simulink model "simulering_ROV_DP_model2"  (R2020a)
settings: Solver=VariableStepAuto  StartTime=0.0  StopTime=t_sim  RelTol=1e-3
values from neighbouring files (symbols this model uses):
  B_aug = [b11 b12 b13 b14 b15 b16 ... (first row only)    [constants.m]
  B_psinv_aug = B_aug'/(B_aug*B_aug')    [constants.m]
  coriolis_effect = 1    [run_simulation.m]    (also in run_simulation_STA_controller.m; run_simulation_dp_model.m)
  d_11 = 250    [constants.m]    (also in constants_dp_model.m; constants_model_coriolis.m; constants_process_model.m)
  d_22 = 200    [constants.m]    (also in constants_dp_model.m; constants_model_coriolis.m; constants_process_model.m)
  d_33 = 175    [constants.m]    (also in constants_dp_model.m; constants_model_coriolis.m; constants_process_model.m)
  d_66 = 15    [constants.m]    (also in constants_process_model.m)
  d_n11 = 350    [constants.m]
  d_n22 = 350    [constants.m]
  d_n33 = 400    [constants.m]
  d_n66 = 75    [constants.m]
  Delta = 25    [plot_simulation_feedback.m]    (also in run_simulation.m; run_simulation_SM_controller.m; run_simulation_STA_controller.m; run_simulation_dp_model.m)
  g_z = 9.81    [run_simulation_FL_controller.m]    (also in run_simulation_PID_controller.m = 0.91; run_simulation_SM_controller.m = 0.91; run_simulation_STA_controller.m = 0.91; run_simulation_dp_model.m = 0.91)
  gamma1 = 50    [run_simulation_dp_model.m]    (also in tuning_dp_model.m = 5)
  gamma2 = 35    [run_simulation_dp_model.m]    (also in tuning_dp_model.m = 3.5)
  gamma_e1 = 0.05    [tuning_dp_model.m]
  gamma_e2 = 0.05    [tuning_dp_model.m]
  gamma_e3 = 0.05    [tuning_dp_model.m]
  k_d_psi = 2*m_44*zeta_d_psi*wn_psi-d_44    [run_simulation_PID_controller.m]    (also in run_simulation_SM_controller.m = 10; run_simulation_dp_model.m = 2*m_66*zeta_d_psi*wn_psi-d_66; run_simulation_feedback_linearizing.m = (2*1*k_p_psi*1-d33/(m_A33+m_RB33)); tuning_PID_controller.m = 2*m_66*zeta_d_psi*wn_psi-d_66)
  k_d_z = 30    [run_simulation_SM_controller.m]    (also in run_simulation_dp_model.m = 2*m_33*zeta_d_heave*wn_heave-d_33; tuning_FL_controller.m = 2*m_33*zeta_d_heave*wn_heave-d_33; tuning_SM_controller.m; tuning_dp_model.m = 2*m_33*zeta_d_heave*wn_heave-d_33)
  k_i_z = wn_heave/10*k_p_z    [run_simulation_PID_controller.m]    (also in run_simulation_dp_model.m = wn_heave/50*k_p_z; tuning_FL_controller.m = wn_heave/50*k_p_z; tuning_PID_controller.m = wn_heave/50*k_p_z; tuning_dp_model.m = wn_heave/50*k_p_z)
  k_p_psi = wn_psi^2-lambda*k_p_r    [run_simulation_FL_controller.m]    (also in run_simulation_PID_controller.m = wn_psi^2*m_44; run_simulation_dp_model.m = wn_psi^2*m_66; run_simulation_feedback_linearizing.m = tau_r_max/deg2rad(45); run_simulation_feedback_linearizing_second_try.m = wn_psi^2*m_44)
  k_p_u = m_11*pole_u-d_11    [run_simulation_FL_controller.m]    (also in run_simulation_PID_controller.m = 10; run_simulation_dp_model.m = pole_u-d_11/m_11; run_simulation_feedback_linearizing.m = tau_u_max/100; run_simulation_feedback_linearizing_second_try.m = 1)
  k_p_v = m_22*pole_v-d_22    [run_simulation_FL_controller.m]    (also in run_simulation_PID_controller.m = 10; run_simulation_dp_model.m = pole_v-d_22/m_22; run_simulation_feedback_linearizing.m = tau_v_max/100; run_simulation_feedback_linearizing_second_try.m = 1)
  k_p_z = wn_heave^2*m_33    [run_simulation_PID_controller.m]    (also in run_simulation_dp_model.m; tuning_FL_controller.m; tuning_PID_controller.m; tuning_dp_model.m)
  m_11 = m_RB11+m_A11    (= 144)    [constants.m]    (also in constants_dp_model.m; constants_model_coriolis.m; constants_process_model.m)
  m_22 = m_RB22+m_A22    (= 162)    [constants.m]    (also in constants_dp_model.m; constants_model_coriolis.m; constants_process_model.m)
  m_66 = m_RB66+m_A66    (= 18.2)    [constants.m]    (also in constants_process_model.m)
  m_A11 = 54    [constants.m]    (also in constants_dp_model.m; constants_model_coriolis.m; constants_process_model.m)
  m_A22 = 72    [constants.m]    (also in constants_dp_model.m; constants_model_coriolis.m; constants_process_model.m)
  m_A33 = 360    [constants.m]    (also in constants_dp_model.m; constants_model_coriolis.m; constants_process_model.m)
  m_A66 = 5.2    [constants.m]    (also in constants_process_model.m)
  m_RB11 = 90    [constants.m]    (also in constants_dp_model.m; constants_model_coriolis.m; constants_process_model.m)
  m_RB22 = 90    [constants.m]    (also in constants_dp_model.m; constants_model_coriolis.m; constants_process_model.m)
  m_RB33 = 90    [constants.m]    (also in constants_dp_model.m; constants_model_coriolis.m; constants_process_model.m)
  m_RB66 = 13    [constants.m]    (also in constants_process_model.m)
  N_nodes = N_elements +1    (= 1001)    [plot_simulation_dp.m]    (also in plot_simulation_feedback.m)
  nonlinear_damping = 0    [run_simulation.m]    (also in run_simulation_STA_controller.m = 1; run_simulation_dp_model.m = 1)
  omega_ref = 1.5    [run_simulation.m]    (also in run_simulation_FL_controller.m = 0.4; run_simulation_PID_controller.m = 0.4; run_simulation_SM_controller.m; run_simulation_STA_controller.m)
  psi0 = deg2rad(psi0)    [constants.m]    (also in constants_dp_model.m; constants_model_coriolis.m; constants_process_model.m)
  psi_r = deg2rad(-45)    [run_simulation.m]    (also in run_simulation_SM_controller.m; run_simulation_STA_controller.m; run_simulation_dp_model.m)
  psi_r1 = deg2rad(psi_r1)    [run_simulation.m]    (also in run_simulation_FL_controller.m = 45; run_simulation_PID_controller.m = 45; run_simulation_SM_controller.m; run_simulation_STA_controller.m)
  psi_r2 = deg2rad(psi_r2)    [run_simulation.m]    (also in run_simulation_FL_controller.m = 90; run_simulation_PID_controller.m = 90; run_simulation_SM_controller.m; run_simulation_STA_controller.m)
  r0 = 0    [constants.m]    (also in constants_dp_model.m; constants_model_coriolis.m; constants_process_model.m)
  step_response = 1    [plot_simulation_feedback.m]    (also in run_simulation.m; run_simulation_SM_controller.m; run_simulation_STA_controller.m; run_simulation_dp_model.m)
  T_ref = 0.2    [run_simulation.m]    (also in run_simulation_FL_controller.m; run_simulation_PID_controller.m; run_simulation_SM_controller.m; run_simulation_STA_controller.m)
  tau_r_max = sqrt(torque_co'*torque_co)    [constants.m]    (also in constants_dp_model.m; constants_model_coriolis.m; constants_process_model.m; run_simulation_feedback_linearizing.m = sqrt(torque_co'*torque_co)/(m_A33+m_RB33))
  tau_u_max = (F_max*cos(alpha1)+F_max*cos(alpha2)+F_max*cos(alpha3)+F_max*cos(alpha4))    [constants.m]    (also in constants_dp_model.m; constants_model_coriolis.m; constants_process_model.m; run_simulation_feedback_linearizing.m = (F_max*cos(alpha1)+F_max*cos(alpha2)+F_max*cos(alpha3)+F_max)
  tau_v_max = (F_max*sin(alpha1)-F_max*sin(alpha2)+F_max*sin(alpha3)-F_max*sin(alpha4))    [constants.m]    (also in constants_dp_model.m; constants_model_coriolis.m; constants_process_model.m; run_simulation_feedback_linearizing.m = (F_max*sin(alpha1)-F_max*sin(alpha2)+F_max*sin(alpha3)-F_max)
  tau_w_max = 2*F_max    (= 240)    [constants.m]    (also in constants_dp_model.m; constants_model_coriolis.m; constants_process_model.m)
  time_step = 700    [run_simulation.m]    (also in run_simulation_SM_controller.m; run_simulation_STA_controller.m; run_simulation_dp_model.m)
  u0 = 0    [constants.m]    (also in constants_dp_model.m; constants_model_coriolis.m; constants_process_model.m)
  u_r = 0.14    [run_simulation.m]    (also in run_simulation_FL_controller.m = 0.2; run_simulation_PID_controller.m = 0.2; run_simulation_SM_controller.m; run_simulation_STA_controller.m)
  v0 = 0    [constants.m]    (also in constants_dp_model.m; constants_model_coriolis.m; constants_process_model.m)
  v_r = 0.14    [run_simulation.m]    (also in run_simulation_FL_controller.m = 0; run_simulation_PID_controller.m = 0; run_simulation_SM_controller.m; run_simulation_STA_controller.m)
  w0 = 0    [constants.m]    (also in constants_dp_model.m; constants_model_coriolis.m; constants_process_model.m)
  x0 = -2*50    (= -100)    [constants.m]    (also in constants_dp_model.m = 0; constants_model_coriolis.m = 0; constants_process_model.m = 0)
  y0 = 0    [constants.m]    (also in constants_dp_model.m; constants_model_coriolis.m; constants_process_model.m)
  z0 = 0    [constants.m]    (also in constants_dp_model.m; constants_model_coriolis.m; constants_process_model.m)
  z_r = 10    [run_simulation.m]    (also in run_simulation_FL_controller.m = 1; run_simulation_PID_controller.m = 1; run_simulation_SM_controller.m; run_simulation_STA_controller.m)
  zeta_ref = 1    [run_simulation.m]    (also in run_simulation_FL_controller.m; run_simulation_PID_controller.m; run_simulation_SM_controller.m; run_simulation_STA_controller.m)
undefined symbols (not defined in the file or in its folder): alpha_k, radius_lim, waypoints
(part 1 of 2)
settings Model: SimulationMode=rapid-accelerator  Creator=kenng  LastModifiedBy=kenng

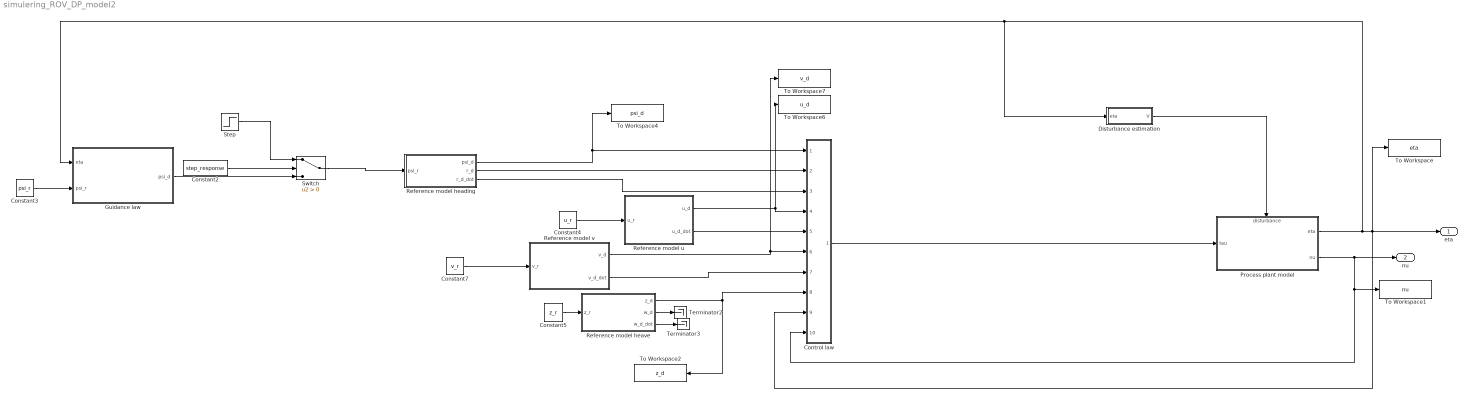
== system simulering_ROV_DP_model2 ==
  Constant2 : Constant  Value=step_response
  Constant3 : Constant  Value=psi_r
  Constant4 : Constant  Value=u_r
  Constant5 : Constant  Value=z_r
  Constant7 : Constant  Value=v_r
  Control law : Subsystem
  Disturbance estimation : Subsystem
  Guidance law : Subsystem
  Process plant model : Subsystem
      settings: PortSchema="{\"entries\":[{\"content\":{\"sides\":[{\"content\":{\"connectorIds\":[\"In1\"]},\"type\":\"ConnectorPlacement.EquallySpacedRectSide\",\"uuid\":\"e717a587-3200-458e-ba24-dd41565550b9\"},{\"content\":{\"connectorIds\":[\"Out1\",\"Out2\"],\"side\":\"RIGHT\"},\"type\":\"ConnectorPlacement.EquallySpacedRectSide\",\"uuid\":\"302c9cc9-c34e-45c2-bf93-40982187bd66\"},{\"content\":{\"connectorIds\":[\"In2\"],\"side\":\"TOP\"},\"type\":\"ConnectorPlacement.EquallySpacedRectSide\",\"uuid\":\"4b1c13ad-6fa1-447d-8a08-ad292496a8ea\"}]},\"type\":\"ConnectorPlacement.EquallySpacedConnector\",\"uuid\":\"78ff5622-69b9-4402-ac71-5e2cc2861626\"}],\"packageUris\":[\"http://schema.mathworks.com/mf0/Connector/19700101\"],\"version\":\"1.0\"}"
  Reference model heading : Subsystem
  Reference model heave : Subsystem
  Reference model u : Subsystem
  Reference model v : Subsystem
  Step : Step  Time=time_step  Before=psi_r1  After=psi_r2  SampleTime=0
  Switch : Switch  Criteria=u2 > Threshold
  Terminator2 : Terminator
  Terminator3 : Terminator
  To Workspace : ToWorkspace  VariableName=eta  SaveFormat=Structure With Time  SampleTime=-1
  To Workspace1 : ToWorkspace  VariableName=nu  SaveFormat=Structure With Time  SampleTime=-1
  To Workspace2 : ToWorkspace  VariableName=z_d  SaveFormat=Structure With Time  SampleTime=-1
  To Workspace4 : ToWorkspace  VariableName=psi_d  SaveFormat=Structure With Time  SampleTime=-1
  To Workspace6 : ToWorkspace  VariableName=u_d  SaveFormat=Structure With Time  SampleTime=-1
  To Workspace7 : ToWorkspace  VariableName=v_d  SaveFormat=Structure With Time  SampleTime=-1
  eta : Outport
  nu : Outport  Port=2
  wires:
  Disturbance estimation/1(V) -> Process plant model/2(disturbance)
  Reference model heave/1(z_d) -> Control law/8(z_d), To Workspace2/1
  Process plant model/2(nu) -> nu/1, To Workspace1/1, Control law/10(nu_aug)
  Reference model heading/2(r_d) -> Control law/2(r_d)
  Process plant model/1(eta) -> Disturbance estimation/1(eta), Guidance law/1(eta), To Workspace/1, Control law/9(eta_aug), eta/1
  Constant4/1 -> Reference model u/1(u_r)
  Reference model heave/3(w_d_dot) -> Terminator3/1
  Reference model heading/3(r_d_dot) -> Control law/3(r_d_dot)
  Constant3/1 -> Guidance law/2(psi_r)
  Reference model v/1(v_d) -> To Workspace7/1, Control law/6(v_d)
  Constant7/1 -> Reference model v/1(v_r)
  Constant2/1 -> Switch/2
  Step/1 -> Switch/1
  Reference model heading/1(psi_d) -> To Workspace4/1, Control law/1(psi_d)
  Guidance law/1(psi_d) -> Switch/3
  Reference model u/2(u_d_dot) -> Control law/5(u_d_dot)
  Reference model v/2(v_d_dot) -> Control law/7(v_d_dot)
  Reference model u/1(u_d) -> To Workspace6/1, Control law/4(u_d)
  Constant5/1 -> Reference model heave/1(z_r)
  Control law/1(tau) -> Process plant model/1(tau)
  Switch/1 -> Reference model heading/1(psi_r)
  Reference model heave/2(w_d) -> Terminator2/1

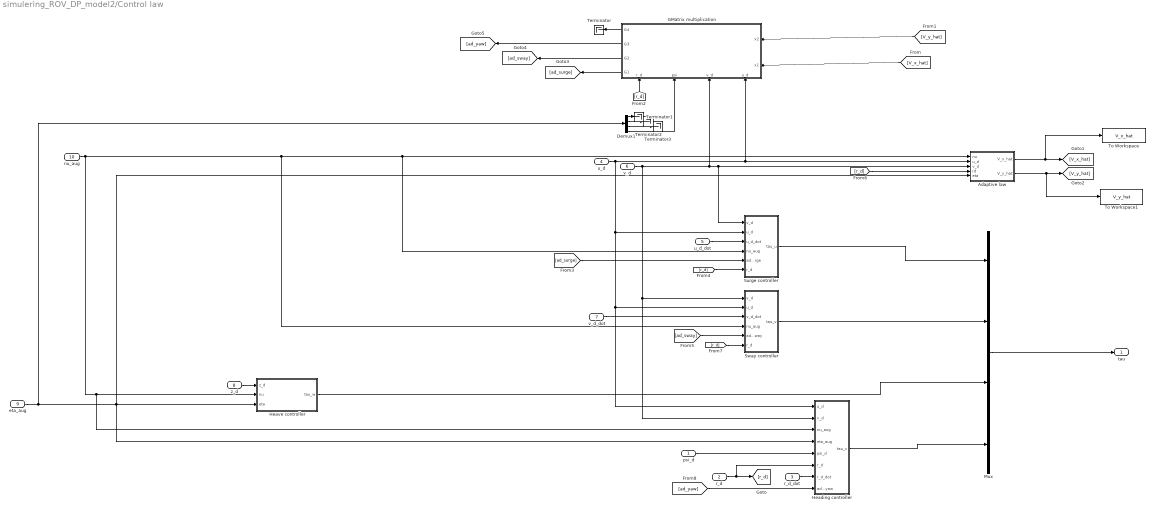
== system simulering_ROV_DP_model2/Control law ==
  psi_d : Inport
  r_d : Inport  Port=2
  r_d_dot : Inport  Port=3
  u_d : Inport  Port=4
  u_d_dot : Inport  Port=5
  v_d : Inport  Port=6
  v_d_dot : Inport  Port=7
  z_d : Inport  Port=8
  eta_aug : Inport  Port=9
  nu_aug : Inport  Port=10
  Adaptive law : Subsystem
  Demux1 : Demux
  GMatrix multiplication : Subsystem
      settings: PortSchema="{\"entries\":[{\"content\":{\"sides\":[{\"content\":{\"connectorIds\":[\"In1\",\"In2\"]},\"type\":\"ConnectorPlacement.EquallySpacedRectSide\",\"uuid\":\"9ba4c88d-ea64-4839-ba97-30354f13a45d\"},{\"content\":{\"connectorIds\":[\"Out1\",\"Out2\",\"Out3\",\"Out4\"],\"side\":\"RIGHT\"},\"type\":\"ConnectorPlacement.EquallySpacedRectSide\",\"uuid\":\"725c894e-5f8f-4bae-9932-022004f91ed5\"},{\"content\":{\"connectorIds\":[\"In3\",\"In4\",\"In5\",\"In6\"],\"side\":\"TOP\"},\"type\":\"ConnectorPlacement.EquallySpacedRectSide\",\"uuid\":\"1baacd43-df16-490e-9b65-a9d644f3ef45\"}]},\"type\":\"ConnectorPlacement.EquallySpacedConnector\",\"uuid\":\"5a604f41-3831-4815-89f9-d7d0823191fd\"}],\"packageUris\":[\"http://schema.mathworks.com/mf0/Connector/19700101\"],\"version\":\"1.0\"}"
  Heading controller : Subsystem
  Heave controller : Subsystem
  Mux : Mux
  Surge controller : Subsystem
  Sway controller : Subsystem
  Terminator{,1..3} (4 alike) : Terminator
  To Workspace : ToWorkspace  VariableName=V_x_hat  SaveFormat=Structure With Time  SampleTime=-1
  To Workspace1 : ToWorkspace  VariableName=V_y_hat  SaveFormat=Structure With Time  SampleTime=-1
  tau : Outport
  wires:
  Heave controller/1(tau_w) -> Mux/3
  Mux/1 -> tau/1
  nu_aug/1 -> Heading controller/3(nu_aug), Heave controller/2(nu), Sway controller/4(nu_aug), Surge controller/4(nu_aug), Adaptive law/1(nu)
  eta_aug/1 -> Demux1/1, Heading controller/4(eta_aug), Heave controller/3(eta), Adaptive law/5(eta)
  u_d/1 -> Surge controller/2(u_d), Heading controller/1(u_d), Sway controller/2(u_d), GMatrix multiplication/3(u_d), Adaptive law/2(u_d)
  v_d/1 -> Sway controller/1(v_d), Heading controller/2(v_d), GMatrix multiplication/4(v_d), Surge controller/1(v_d), Adaptive law/3(v_d)
  Adaptive law/1(V_x_hat) -> To Workspace/1, [V_x_hat]
  Adaptive law/2(V_y_hat) -> To Workspace1/1, [V_y_hat]
  z_d/1 -> Heave controller/1(z_d)
  r_d/1 -> Heading controller/6(r_d), [r_d]
  [r_d] -> Adaptive law/4(rd)
  GMatrix multiplication/4(G4) -> Terminator/1
  [V_x_hat] -> GMatrix multiplication/1(x1)
  [V_y_hat] -> GMatrix multiplication/2(x2)
  Demux1/4 -> GMatrix multiplication/5(psi)
  Demux1/1 -> Terminator1/1
  Demux1/2 -> Terminator2/1
  Demux1/3 -> Terminator3/1
  [r_d] -> GMatrix multiplication/6(r_d)
  GMatrix multiplication/3(G3) -> [ad_yaw]
  GMatrix multiplication/2(G2) -> [ad_sway]
  GMatrix multiplication/1(G1) -> [ad_surge]
  u_d_dot/1 -> Surge controller/3(u_d_dot)
  [ad_surge] -> Surge controller/5(adaptive_surge)
  [r_d] -> Surge controller/6(r_d)
  [ad_sway] -> Sway controller/5(adaptive_sway)
  [r_d] -> Sway controller/6(r_d)
  v_d_dot/1 -> Sway controller/3(v_d_dot)
  Sway controller/1(tau_v) -> Mux/2
  Surge controller/1(tau_u) -> Mux/1
  Heading controller/1(tau_v) -> Mux/4
  r_d_dot/1 -> Heading controller/7(r_d_dot)
  psi_d/1 -> Heading controller/5(psi_d)
  [ad_yaw] -> Heading controller/8(adaptive_yaw)

== system simulering_ROV_DP_model2/Disturbance estimation ==
  note: Note that u and v are rotated 90 degrees in Lars masters thesis (such that u goes to the right and v er upwards) if we are to follow the NED frame u have to be upwards and v eastwards
  eta : Inport
  2-D Lookup V_x_interp : Lookup_n-D  LookupTableObject=''  BreakpointsForDimension1=[-2*50:2*50]  BreakpointsForDimension2=[-2*50:5*50]  BreakpointsForDimension1FirstPoint=10  BreakpointsForDimension2FirstPoint=10  BreakpointsForDimension1Spacing=12  BreakpointsForDimension2Spacing=12  IndexSearchMethod=Evenly spaced points  Table=V_y_mat'  InterpMethod=Linear Lagrange  ExtrapMethod=Clip  DiagnosticForOutOfRangeInput=Error  InternalRulePriority=Speed  RndMeth=Simplest  InputSameDT=on
  2-D Lookup V_y_interp : Lookup_n-D  LookupTableObject=''  BreakpointsForDimension1=[-2*50:2*50]  BreakpointsForDimension2=[-2*50:5*50]  BreakpointsForDimension1FirstPoint=10  BreakpointsForDimension2FirstPoint=10  BreakpointsForDimension1Spacing=12  BreakpointsForDimension2Spacing=12  IndexSearchMethod=Evenly spaced points  Table=V_x_mat'  InterpMethod=Linear Lagrange  ExtrapMethod=Clip  DiagnosticForOutOfRangeInput=Error  InternalRulePriority=Speed  RndMeth=Simplest  InputSameDT=on
  Demux : Demux
  Mux1 : Mux  Inputs=2
  Terminator : Terminator
  Terminator1 : Terminator
  To Workspace5 : ToWorkspace  VariableName=disturbance  SaveFormat=Structure With Time  SampleTime=-1
  V : Outport
  wires:
  2-D Lookup V_x_interp/1 -> Mux1/1
  eta/1 -> Demux/1
  Mux1/1 -> V/1, To Workspace5/1
  Demux/3 -> Terminator/1
  Demux/1 -> 2-D Lookup V_y_interp/1, 2-D Lookup V_x_interp/1
  2-D Lookup V_y_interp/1 -> Mux1/2
  Demux/2 -> 2-D Lookup V_y_interp/2, 2-D Lookup V_x_interp/2
  Demux/4 -> Terminator1/1

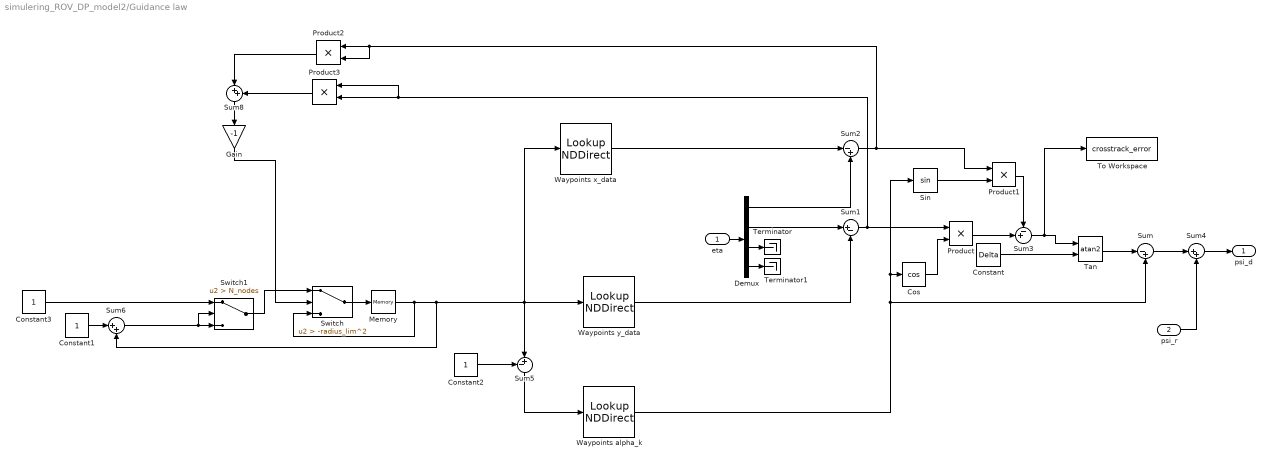
== system simulering_ROV_DP_model2/Guidance law ==
  eta : Inport
  psi_r : Inport  Port=2
  Constant : Constant  Value=Delta
  Constant1 : Constant
  Constant2 : Constant
  Constant3 : Constant
  Cos : Trigonometry  Operator=cos
  Demux : Demux
  Gain : Gain  Gain=-1
  Memory : Memory  InitialCondition=1
  Product{,1..3} (4 alike) : Product
  Sin : Trigonometry
  Sum : Sum  Inputs=|-+
  Sum1 : Sum  Inputs=|+-
  Sum2 : Sum  Inputs=|-+
  Sum3 : Sum  Inputs=-+|
  Sum4 : Sum  Inputs=|++
  Sum5 : Sum  Inputs=-+|
  Sum6 : Sum  Inputs=|++
  Sum8 : Sum  Inputs=|++
  Switch : Switch  Criteria=u2 > Threshold  Threshold=-radius_lim^2
  Switch1 : Switch  Criteria=u2 > Threshold  Threshold=N_nodes
  Tan : Trigonometry  Operator=atan2
  Terminator : Terminator
  Terminator1 : Terminator
  To Workspace : ToWorkspace  VariableName=crosstrack_error  SaveFormat=Structure With Time  SampleTime=-1
  Waypoints alpha_k : LookupNDDirect  NumberOfTableDimensions=1  Table=alpha_k(:, 1)
  Waypoints x_data : LookupNDDirect  NumberOfTableDimensions=1  Table=waypoints(:, 1)
  Waypoints y_data : LookupNDDirect  NumberOfTableDimensions=1  Table=waypoints(:, 2)
  psi_d : Outport
  wires:
  eta/1 -> Demux/1
  Demux/3 -> Terminator/1
  Demux/4 -> Terminator1/1
  Constant/1 -> Tan/2
  Waypoints alpha_k/1 -> Sum/2, Sin/1, Cos/1
  Tan/1 -> Sum/1
  Demux/2 -> Sum1/1
  Cos/1 -> Product/2
  Sum1/1 -> Product/1, Product3/2, Product3/1
  Sin/1 -> Product1/2
  Demux/1 -> Sum2/2
  Sum2/1 -> Product2/2, Product2/1, Product1/1
  Product/1 -> Sum3/2
  Product1/1 -> Sum3/1
  Sum3/1 -> To Workspace/1, Tan/1
  Sum/1 -> Sum4/1
  Sum4/1 -> psi_d/1
  psi_r/1 -> Sum4/2
  Memory/1 -> Switch/3, Waypoints x_data/1, Waypoints y_data/1, Sum5/2, Sum6/2
  Waypoints x_data/1 -> Sum2/1
  Waypoints y_data/1 -> Sum1/2
  Sum5/1 -> Waypoints alpha_k/1
  Switch/1 -> Memory/1
  Constant1/1 -> Sum6/1
  Product2/1 -> Sum8/1
  Product3/1 -> Sum8/2
  Sum8/1 -> Gain/1
  Sum6/1 -> Switch1/3, Switch1/2
  Constant3/1 -> Switch1/1
  Gain/1 -> Switch/2
  Switch1/1 -> Switch/1
  Constant2/1 -> Sum5/1

== system simulering_ROV_DP_model2/Process plant model ==
  note: tau: 4x1 vector = [surge sway heave yaw]^T
  note: Disturbance: 3x1 vector = [Vx Vy gz]^t
  tau : Inport
  disturbance : Inport  Port=2
  Demux : Demux
  Kinematics : Subsystem
  Kinetics : Subsystem
  Terminator : Terminator
  Terminator1 : Terminator
  Terminator2 : Terminator
  Thruster saturation : Subsystem
  To Workspace2 : ToWorkspace  VariableName=tau_unsat  SaveFormat=Structure With Time  SampleTime=-1
  To Workspace3 : ToWorkspace  VariableName=tau_sat  SaveFormat=Structure With Time  SampleTime=-1
  eta : Outport
  nu : Outport  Port=2
  wires:
  Kinetics/1(nu) -> nu/1, Kinematics/1(nu)
  Demux/4 -> Kinetics/3(psi)
  Demux/2 -> Terminator1/1
  Kinematics/1(eta) -> eta/1, Demux/1
  Demux/1 -> Terminator/1
  Demux/3 -> Terminator2/1
  disturbance/1 -> Kinetics/1(disturbance)
  Thruster saturation/1(tau_sat) -> Kinetics/2(tau), To Workspace3/1
  tau/1 -> Thruster saturation/1(tau_unsat), To Workspace2/1

== system simulering_ROV_DP_model2/Reference model heading ==
  note: psi_r
  note: psi_d
  note: r_d
  note: a_d
  psi_r : Inport
  Gain : Gain  Gain=(2*zeta_ref+1)*omega_ref
  Gain1 : Gain  Gain=(2*zeta_ref+1)*omega_ref^2
  Gain2 : Gain  Gain=omega_ref^3
  Integrator : Integrator  InitialCondition=r0
  Integrator1 : Integrator
  Integrator2 : Integrator  InitialCondition=psi0
  Saturation : Saturate  UpperLimit=tau_r_max/(m_RB11*0.2^2)  LowerLimit=-tau_r_max/(m_RB11*0.2^2)
  Sum : Sum  Inputs=|+-
  Sum1 : Sum  Inputs=-+|
  Sum2 : Sum  Inputs=-+|
  psi_d : Outport
  r_d : Outport  Port=2
  r_d_dot : Outport  Port=3
  wires:
  Sum1/1 -> Integrator1/1
  Sum2/1 -> Gain2/1
  Integrator2/1 -> psi_d/1, Sum2/1
  Sum/1 -> Sum1/2
  Saturation/1 -> Gain/1, Integrator/1, r_d_dot/1
  Integrator/1 -> r_d/1, Gain1/1, Integrator2/1
  Gain2/1 -> Sum/1
  Gain/1 -> Sum/2
  Gain1/1 -> Sum1/1
  Integrator1/1 -> Saturation/1
  psi_r/1 -> Sum2/2

== system simulering_ROV_DP_model2/Reference model heave ==
  note: w_d_dot
  note: z_r
  note: z_d
  note: w_d
  note: a_ud
  z_r : Inport
  Gain : Gain  Gain=(2*zeta_ref+1)*omega_ref
  Gain1 : Gain  Gain=(2*zeta_ref+1)*omega_ref^2
  Gain2 : Gain  Gain=omega_ref^3
  Integrator : Integrator  InitialCondition=w0
  Integrator1 : Integrator
  Integrator2 : Integrator  InitialCondition=z0
  Saturation : Saturate  UpperLimit=tau_w_max/m_RB11  LowerLimit=-tau_w_max/m_RB11
  Sum : Sum  Inputs=|+-
  Sum1 : Sum  Inputs=-+|
  Sum2 : Sum  Inputs=-+|
  z_d : Outport
  w_d : Outport  Port=2
  w_d_dot : Outport  Port=3
  wires:
  Sum1/1 -> Integrator1/1
  Sum2/1 -> Gain2/1
  Integrator2/1 -> z_d/1, Sum2/1
  Sum/1 -> Sum1/2
  Saturation/1 -> Integrator/1, w_d_dot/1, Gain/1
  Gain2/1 -> Sum/1
  Gain/1 -> Sum/2
  Gain1/1 -> Sum1/1
  Integrator1/1 -> Saturation/1
  z_r/1 -> Sum2/2
  Integrator/1 -> w_d/1, Gain1/1, Integrator2/1

== system simulering_ROV_DP_model2/Reference model u ==
  note: u_r
  u_r : Inport
  Gain : Gain  Gain=1/T_ref
  Integrator : Integrator  InitialCondition=u0
  Saturation : Saturate  UpperLimit=tau_u_max/m_RB11  LowerLimit=-tau_u_max/m_RB11
  Sum : Sum  Inputs=|+-
  u_d : Outport
  u_d_dot : Outport  Port=2
  wires:
  u_r/1 -> Sum/1
  Sum/1 -> Gain/1
  Integrator/1 -> u_d/1, Sum/2
  Gain/1 -> Saturation/1
  Saturation/1 -> u_d_dot/1, Integrator/1

== system simulering_ROV_DP_model2/Reference model v ==
  note: v_r
  v_r : Inport
  Gain : Gain  Gain=1/T_ref
  Integrator : Integrator  InitialCondition=v0
  Saturation1 : Saturate  UpperLimit=tau_v_max/m_RB11  LowerLimit=-tau_v_max/m_RB11
  Sum : Sum  Inputs=|+-
  v_d : Outport
  v_d_dot : Outport  Port=2
  wires:
  v_r/1 -> Sum/1
  Sum/1 -> Gain/1
  Gain/1 -> Saturation1/1
  Saturation1/1 -> v_d_dot/1, Integrator/1
  Integrator/1 -> v_d/1, Sum/2

== system simulering_ROV_DP_model2/Control law/Adaptive law ==
  note: last element is 0 regardless so does not need to send in signal. But in theory it should have been psi tilde times kpsi and times 2 going in for x4
  nu : Inport
  u_d : Inport  Port=2
  v_d : Inport  Port=3
  rd : Inport  Port=4
  eta : Inport  Port=5
  "\"2*kp_psi*psi tilde\"" : Constant  Value=0
  Demux : Demux
  Demux1 : Demux
  GMatrix transpose multiplication : Subsystem
      settings: PortSchema="{\"entries\":[{\"content\":{\"sides\":[{\"content\":{\"connectorIds\":[\"In1\",\"In2\",\"In3\",\"In4\"]},\"type\":\"ConnectorPlacement.EquallySpacedRectSide\",\"uuid\":\"9ba4c88d-ea64-4839-ba97-30354f13a45d\"},{\"content\":{\"connectorIds\":[\"Out1\",\"Out2\"],\"side\":\"RIGHT\"},\"type\":\"ConnectorPlacement.EquallySpacedRectSide\",\"uuid\":\"725c894e-5f8f-4bae-9932-022004f91ed5\"},{\"content\":{\"connectorIds\":[\"In5\",\"In6\",\"In7\",\"In8\"],\"side\":\"TOP\"},\"type\":\"ConnectorPlacement.EquallySpacedRectSide\",\"uuid\":\"1baacd43-df16-490e-9b65-a9d644f3ef45\"}]},\"type\":\"ConnectorPlacement.EquallySpacedConnector\",\"uuid\":\"5a604f41-3831-4815-89f9-d7d0823191fd\"}],\"packageUris\":[\"http://schema.mathworks.com/mf0/Connector/19700101\"],\"version\":\"1.0\"}"
  Gain : Gain  Gain=gamma1
  Gain1 : Gain  Gain=gamma2
  Gain2 : Gain  Gain=m_11
  Gain3 : Gain  Gain=m_22
  Gain4 : Gain  Gain=m_66
  Integrator : Integrator
  Integrator1 : Integrator
  Sum : Sum  Inputs=-+|
  Sum1 : Sum  Inputs=-+|
  Sum2 : Sum  Inputs=-+|
  Terminator{,1..3} (4 alike) : Terminator
  V_x_hat : Outport
  V_y_hat : Outport  Port=2
  wires:
  GMatrix transpose multiplication/2(GT2) -> Gain1/1
  u_d/1 -> GMatrix transpose multiplication/5(u_d), Sum/1
  v_d/1 -> GMatrix transpose multiplication/6(v_d), Sum1/1
  rd/1 -> GMatrix transpose multiplication/8(r_d), Sum2/1
  Demux/1 -> Sum/2
  Sum/1 -> Gain2/1
  Sum1/1 -> Gain3/1
  Demux/2 -> Sum1/2
  Demux/3 -> Terminator/1
  Demux/4 -> Sum2/2
  Sum2/1 -> Gain4/1
  nu/1 -> Demux/1
  "\"2*kp_psi*psi tilde\""/1 -> GMatrix transpose multiplication/4(x4)
  GMatrix transpose multiplication/1(GT1) -> Gain/1
  Gain1/1 -> Integrator1/1
  Gain2/1 -> GMatrix transpose multiplication/1(x1)
  Gain3/1 -> GMatrix transpose multiplication/2(x2)
  Gain4/1 -> GMatrix transpose multiplication/3(x3)
  Demux1/1 -> Terminator1/1
  Demux1/2 -> Terminator2/1
  Demux1/3 -> Terminator3/1
  eta/1 -> Demux1/1
  Demux1/4 -> GMatrix transpose multiplication/7(psi)
  Gain/1 -> Integrator/1
  Integrator/1 -> V_x_hat/1
  Integrator1/1 -> V_y_hat/1

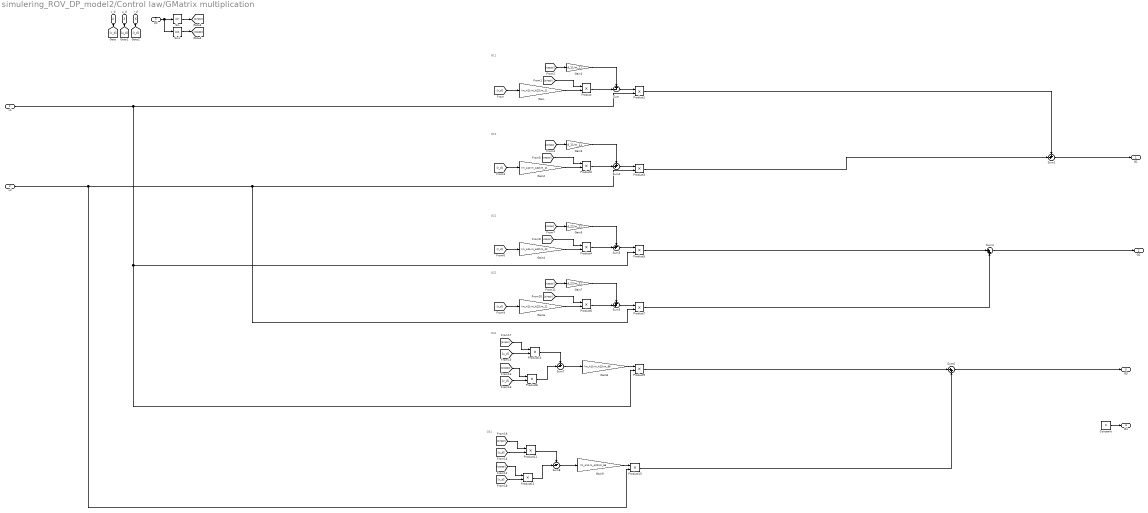
== system simulering_ROV_DP_model2/Control law/GMatrix multiplication ==
  note: G31
  note: G22
  note: G21
  note: G12
  note: G11
  note: G31
  x1 : Inport
  x2 : Inport  Port=2
  u_d : Inport  Port=3
  v_d : Inport  Port=4
  psi : Inport  Port=5
  r_d : Inport  Port=6
  Constant : Constant  Value=0
  Gain : Gain  Gain=(m_A11-m_A22)/m_11
  Gain1 : Gain  Gain=d_11/m_11
  Gain2 : Gain  Gain=(m_A11-m_A22)/m_11
  Gain3 : Gain  Gain=d_11/m_11
  Gain4 : Gain  Gain=(m_A11-m_A22)/m_22
  Gain5 : Gain  Gain=d_22/m_22
  Gain6 : Gain  Gain=(m_A11-m_A22)/m_22
  Gain7 : Gain  Gain=d_22/m_22
  Gain8 : Gain  Gain=(m_A11-m_A22)/m_66
  Gain9 : Gain  Gain=(m_A11-m_A22)/m_66
  Product{,1..13} (14 alike) : Product
  Sin : Trigonometry
  Sin1 : Trigonometry  Operator=cos
  Sum : Sum  Inputs=+-|
  Sum1 : Sum  Inputs=++|
  Sum2 : Sum  Inputs=++|
  Sum3 : Sum  Inputs=-+|
  Sum4 : Sum  Inputs=|++
  Sum5 : Sum  Inputs=++|
  Sum6 : Sum  Inputs=|++
  Sum7 : Sum  Inputs=+-|
  Sum8 : Sum  Inputs=--|
  G1 : Outport
  G2 : Outport  Port=2
  G3 : Outport  Port=3
  G4 : Outport  Port=4
  wires:
  v_d/1 -> [v_d]
  u_d/1 -> [u_d]
  r_d/1 -> [r_d]
  psi/1 -> Sin1/1, Sin/1
  Sin/1 -> [sinpsi]
  Sin1/1 -> [cospsi]
  Product1/1 -> Sum1/1
  Sum/1 -> Product1/1
  Product/1 -> Sum/2
  [r_d] -> Gain/1
  Gain/1 -> Product/2
  [sinpsi] -> Product/1
  [cospsi] -> Gain1/1
  Gain1/1 -> Sum/1
  Product3/1 -> Sum1/2
  Sum1/1 -> G1/1
  Sum2/1 -> Product3/1
  Product2/1 -> Sum2/2
  [r_d] -> Gain2/1
  Gain2/1 -> Product2/2
  [cospsi] -> Product2/1
  [sinpsi] -> Gain3/1
  Gain3/1 -> Sum2/1
  Product5/1 -> Sum4/1
  x1/1 -> Product9/2, Product5/2, Product1/2
  Sum3/1 -> Product5/1
  Product4/1 -> Sum3/2
  [r_d] -> Gain4/1
  Gain4/1 -> Product4/2
  [cospsi] -> Product4/1
  [sinpsi] -> Gain5/1
  Gain5/1 -> Sum3/1
  Sum4/1 -> G2/1
  Product7/1 -> Sum4/2
  Sum5/1 -> Product7/1
  Product6/1 -> Sum5/2
  [r_d] -> Gain6/1
  Gain6/1 -> Product6/2
  [sinpsi] -> Product6/1
  [cospsi] -> Gain7/1
  Gain7/1 -> Sum5/1
  Sum7/1 -> Gain8/1
  [u_d] -> Product10/2
  [sinpsi] -> Product10/1
  [v_d] -> Product8/2
  [cospsi] -> Product8/1
  Product8/1 -> Sum7/2
  Product10/1 -> Sum7/1
  Gain8/1 -> Product9/1
  Product9/1 -> Sum6/1
  Sum6/1 -> G3/1
  Sum8/1 -> Gain9/1
  Product12/1 -> Sum8/2
  Product13/1 -> Sum6/2
  [u_d] -> Product11/2
  x2/1 -> Product13/2, Product7/2, Product3/2
  [sinpsi] -> Product11/1
  [v_d] -> Product12/2
  Gain9/1 -> Product13/1
  [cospsi] -> Product12/1
  Product11/1 -> Sum8/1
  Constant/1 -> G4/1

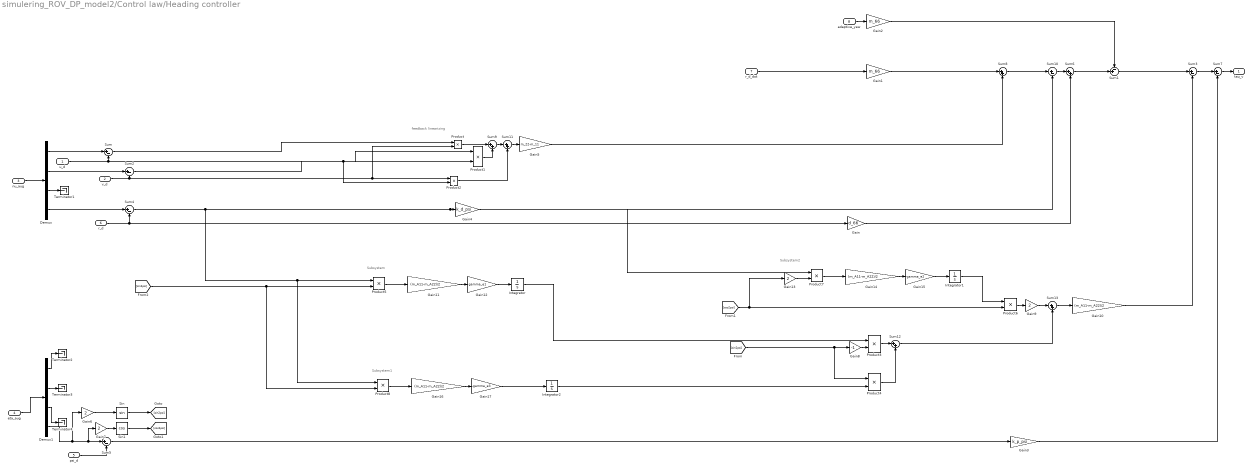
== system simulering_ROV_DP_model2/Control law/Heading controller ==
  note: Subsystem1
  note: Subsystem2
  note: Subsystem
  note: feedback linearizing
  u_d : Inport
  v_d : Inport  Port=2
  nu_aug : Inport  Port=3
  eta_aug : Inport  Port=4
  psi_d : Inport  Port=5
  r_d : Inport  Port=6
  r_d_dot : Inport  Port=7
  adaptive_yaw : Inport  Port=8
  Demux : Demux
  Demux1 : Demux
  Gain : Gain  Gain=d_66
  Gain1 : Gain  Gain=m_66
  Gain{10..11,14,16} (4 alike) : Gain  Gain=(m_A11-m_A22)/2
  Gain12 : Gain  Gain=gamma_e1
  Gain{6..7,9,13} (4 alike) : Gain  Gain=2
  Gain15 : Gain  Gain=-gamma_e2
  Gain17 : Gain  Gain=-gamma_e3
  Gain2 : Gain  Gain=m_66
  Gain3 : Gain  Gain=k_p_psi
  Gain4 : Gain  Gain=k_d_psi
  Gain5 : Gain  Gain=m_22-m_11
  Gain8 : Gain  Gain=-1
  Integrator : Integrator
  Integrator1 : Integrator
  Integrator2 : Integrator
  Product{,1..8} (9 alike) : Product
  Sin : Trigonometry
  Sin1 : Trigonometry  Operator=cos
  Sum{,2..5,7,10} (7 alike) : Sum  Inputs=|+-
  Sum1 : Sum  Inputs=-+|
  Sum{6,8..9,11..13} (6 alike) : Sum  Inputs=|++
  Terminator{1..4} (4 alike) : Terminator
  tau_v : Outport
  wires:
  adaptive_yaw/1 -> Gain2/1
  Gain2/1 -> Sum1/1
  nu_aug/1 -> Demux/1
  Sum1/1 -> Sum3/1
  Sum3/1 -> Sum7/1
  Sum7/1 -> tau_v/1
  Demux/3 -> Terminator1/1
  Demux/1 -> Sum/1
  Demux/2 -> Sum2/1
  Demux/4 -> Sum4/1
  r_d/1 -> Sum4/2, Gain/1
  eta_aug/1 -> Demux1/1
  Demux1/4 -> Gain6/1, Gain7/1, Sum5/1
  psi_d/1 -> Sum5/2
  Demux1/1 -> Terminator2/1
  Demux1/2 -> Terminator3/1
  Demux1/3 -> Terminator4/1
  r_d_dot/1 -> Gain1/1
  Gain/1 -> Sum6/2
  Sum10/1 -> Sum6/1
  Sum8/1 -> Sum10/1
  Sum6/1 -> Sum1/2
  Sum5/1 -> Gain3/1
  Gain3/1 -> Sum7/2
  Gain1/1 -> Sum8/1
  Gain4/1 -> Sum10/2
  Gain5/1 -> Sum8/2
  Sum/1 -> Product/1
  Sum2/1 -> Product1/2
  v_d/1 -> Sum2/2, Product/2, Product2/1
  Sum9/1 -> Sum11/1
  Product2/1 -> Sum11/2
  u_d/1 -> Product2/2, Product1/1, Sum/2
  Product/1 -> Sum9/1
  Product1/1 -> Sum9/2
  Sum11/1 -> Gain5/1
  Sin/1 -> [sin2psi]
  Sin1/1 -> [cos2psi]
  Gain6/1 -> Sin/1
  Gain7/1 -> Sin1/1
  Gain8/1 -> Product3/2
  [sin2psi] -> Product4/1, Gain8/1
  Product3/1 -> Sum12/1
  Product4/1 -> Sum12/2
  Integrator1/1 -> Product6/1
  Product6/1 -> Gain9/1
  Gain9/1 -> Sum13/1
  Sum12/1 -> Sum13/2
  Sum13/1 -> Gain10/1
  Gain10/1 -> Sum3/2
  Integrator/1 -> Product3/1
  Integrator2/1 -> Product4/2
  Product5/1 -> Gain11/1
  Gain11/1 -> Gain12/1
  Gain12/1 -> Integrator/1
  Gain13/1 -> Product7/2
  [cos2psi] -> Gain13/1, Product6/2
  Product7/1 -> Gain14/1
  Gain14/1 -> Gain15/1
  Gain15/1 -> Integrator1/1
  [sin2psi] -> Product8/2, Product5/2
  Sum4/1 -> Product8/1, Product5/1, Product7/1, Gain4/1
  Product8/1 -> Gain16/1
  Gain16/1 -> Gain17/1
  Gain17/1 -> Integrator2/1

== system simulering_ROV_DP_model2/Control law/Heave controller ==
  note: r
  note: psi
  z_d : Inport
  nu : Inport  Port=2
  eta : Inport  Port=3
  Constant : Constant  Value=g_z
  Demux : Demux
  Demux1 : Demux
  Gain : Gain  Gain=k_p_z
  Gain1 : Gain  Gain=k_d_z
  Gain2 : Gain  Gain=k_i_z
  Gain3 : Gain  Gain=-1
  Integrator : Integrator
  Sum : Sum  Inputs=|+-
  Sum1 : Sum  Inputs=|++
  Sum2 : Sum  Inputs=-|+|+
  Terminator{,1,3..4,6..7} (6 alike) : Terminator
  tau_w : Outport
  wires:
  Demux1/2 -> Terminator4/1
  Demux/1 -> Terminator/1
  eta/1 -> Demux/1
  Demux/2 -> Terminator1/1
  Demux1/1 -> Terminator3/1
  Demux/3 -> Sum/1
  nu/1 -> Demux1/1
  Demux1/4 -> Terminator6/1
  Demux/4 -> Terminator7/1
  z_d/1 -> Sum/2
  Sum/1 -> Gain2/1, Gain/1
  Demux1/3 -> Gain1/1
  Gain2/1 -> Integrator/1
  Integrator/1 -> Sum1/1
  Gain/1 -> Sum1/2
  Sum2/1 -> Gain3/1
  Gain3/1 -> tau_w/1
  Gain1/1 -> Sum2/3
  Sum1/1 -> Sum2/2
  Constant/1 -> Sum2/1

== system simulering_ROV_DP_model2/Control law/Surge controller ==
  note: Feedback linearizing
  v_d : Inport
  u_d : Inport  Port=2
  u_d_dot : Inport  Port=3
  nu_aug : Inport  Port=4
  adaptive_surge : Inport  Port=5
  r_d : Inport  Port=6
  Demux : Demux
  Gain : Gain  Gain=m_11
  Gain1 : Gain  Gain=d_11
  Gain2 : Gain  Gain=m_11
  Gain3 : Gain  Gain=k_p_u
  Gain4 : Gain  Gain=-m_22
  Product : Product
  Product1 : Product
  Product2 : Product
  Sum : Sum  Inputs=++|
  Sum1 : Sum  Inputs=-+|
  Sum2 : Sum  Inputs=-+|
  Sum3 : Sum  Inputs=|+-
  Sum4 : Sum  Inputs=|+-
  Sum5 : Sum  Inputs=|++
  Sum6 : Sum  Inputs=|+-
  Sum7 : Sum  Inputs=|++
  Sum8 : Sum  Inputs=|++
  Terminator1 : Terminator
  tau_u : Outport
  wires:
  Gain/1 -> Sum/2
  Gain1/1 -> Sum/1
  u_d_dot/1 -> Gain/1
  u_d/1 -> Sum2/1, Gain1/1
  Sum/1 -> Sum1/2
  adaptive_surge/1 -> Gain2/1
  Gain2/1 -> Sum1/1
  Demux/3 -> Terminator1/1
  nu_aug/1 -> Demux/1
  Demux/1 -> Sum2/2
  Sum1/1 -> Sum3/1
  Sum2/1 -> Gain3/1
  Gain3/1 -> Sum3/2
  Sum3/1 -> Sum7/1
  Sum7/1 -> tau_u/1
  Gain4/1 -> Sum7/2
  Demux/4 -> Sum6/1
  Demux/2 -> Sum4/1
  Product2/1 -> Sum8/2
  Sum8/1 -> Gain4/1
  Sum5/1 -> Sum8/1
  Product1/1 -> Sum5/2
  v_d/1 -> Product2/1, Product1/1, Sum4/2
  Sum6/1 -> Product1/2
  r_d/1 -> Product2/2, Sum6/2, Product/2
  Product/1 -> Sum5/1
  Sum4/1 -> Product/1

== system simulering_ROV_DP_model2/Control law/Sway controller ==
  note: Feedback linearizing
  v_d : Inport
  u_d : Inport  Port=2
  v_d_dot : Inport  Port=3
  nu_aug : Inport  Port=4
  adaptive_sway : Inport  Port=5
  r_d : Inport  Port=6
  Demux : Demux
  Gain : Gain  Gain=m_22
  Gain1 : Gain  Gain=d_22
  Gain2 : Gain  Gain=m_22
  Gain3 : Gain  Gain=k_p_v
  Gain4 : Gain  Gain=m_11
  Product : Product
  Product1 : Product
  Product2 : Product
  Sum : Sum  Inputs=++|
  Sum1 : Sum  Inputs=-+|
  Sum2 : Sum  Inputs=-+|
  Sum3 : Sum  Inputs=|+-
  Sum4 : Sum  Inputs=|+-
  Sum5 : Sum  Inputs=|++
  Sum6 : Sum  Inputs=|+-
  Sum7 : Sum  Inputs=|++
  Sum8 : Sum  Inputs=|++
  Terminator1 : Terminator
  tau_v : Outport
  wires:
  Gain/1 -> Sum/2
  Gain1/1 -> Sum/1
  v_d_dot/1 -> Gain/1
  v_d/1 -> Sum2/1, Gain1/1
  Sum/1 -> Sum1/2
  adaptive_sway/1 -> Gain2/1
  Gain2/1 -> Sum1/1
  Demux/3 -> Terminator1/1
  nu_aug/1 -> Demux/1
  Sum1/1 -> Sum3/1
  Sum2/1 -> Gain3/1
  Gain3/1 -> Sum3/2
  Sum3/1 -> Sum7/1
  Sum7/1 -> tau_v/1
  Gain4/1 -> Sum7/2
  Demux/4 -> Sum6/1
  Product2/1 -> Sum8/2
  Sum8/1 -> Gain4/1
  Sum5/1 -> Sum8/1
  Product1/1 -> Sum5/2
  u_d/1 -> Sum4/2, Product2/1, Product1/1
  r_d/1 -> Product/2, Sum6/2, Product2/2
  Product/1 -> Sum5/1
  Demux/2 -> Sum2/2
  Demux/1 -> Sum4/1
  Sum4/1 -> Product/1
  Sum6/1 -> Product1/2

== system simulering_ROV_DP_model2/Process plant model/Kinematics ==
  nu : Inport
  Cos : Trigonometry  Operator=cos
  Demux : Demux
  Integrator : Integrator  InitialCondition=psi0
  Integrator1 : Integrator  InitialCondition=z0
  Integrator2 : Integrator  InitialCondition=x0
  Integrator3 : Integrator  InitialCondition=y0
  Mux : Mux
  Product{,1..3} (4 alike) : Product
  Sin : Trigonometry
  Sum : Sum  Inputs=|++
  Sum1 : Sum  Inputs=|+-
  eta : Outport
  wires:
  Sin/1 -> [sinpsi]
  Demux/3 -> Integrator1/1
  Demux/1 -> Product1/1, Product/1
  Demux/2 -> Product3/1, Product2/1
  [sinpsi] -> Product3/2
  [psi] -> Sin/1, Cos/1
  [cospsi] -> Product2/2
  Cos/1 -> [cospsi]
  Product1/1 -> Sum/1
  Integrator/1 -> Mux/4, [psi]
  [sinpsi] -> Product1/2
  Product/1 -> Sum1/1
  Sum1/1 -> Integrator2/1
  Demux/4 -> Integrator/1
  Sum/1 -> Integrator3/1
  [cospsi] -> Product/2
  nu/1 -> Demux/1
  Product2/1 -> Sum/2
  Product3/1 -> Sum1/2
  Integrator3/1 -> Mux/2
  Integrator1/1 -> Mux/3
  Integrator2/1 -> Mux/1
  Mux/1 -> eta/1

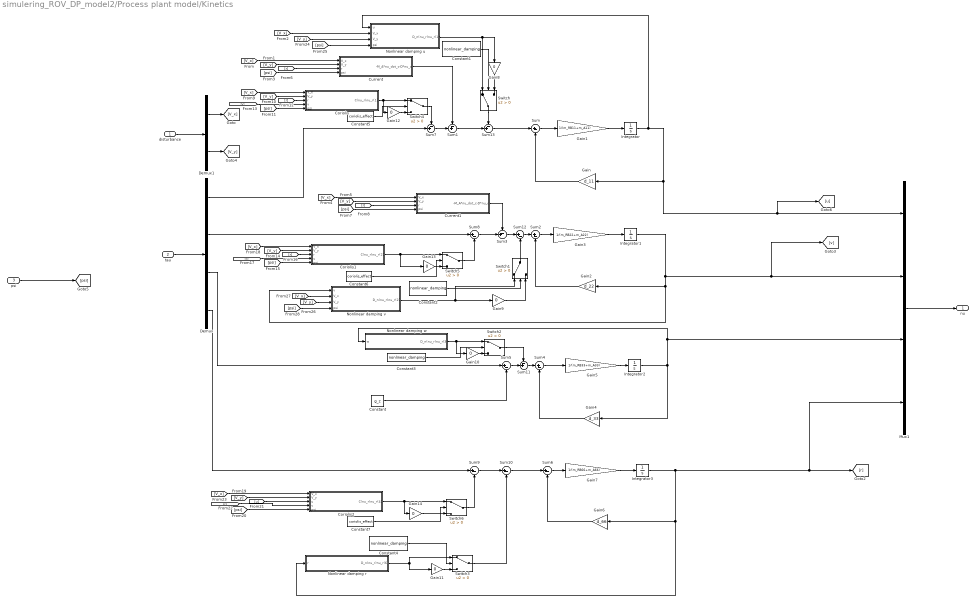
== system simulering_ROV_DP_model2/Process plant model/Kinetics ==
  disturbance : Inport
  tau : Inport  Port=2
  psi : Inport  Port=3
  Constant : Constant  Value=g_z
  Constant{1..4} (4 alike) : Constant  Value=nonlinear_damping
  Constant5 : Constant  Value=coriolis_effect
  Constant6 : Constant  Value=coriolis_effect
  Constant7 : Constant  Value=coriolis_effect
  Coriolis : Subsystem
  Coriolis1 : Subsystem
  Coriolis2 : Subsystem
  Current : Subsystem
  Current1 : Subsystem
  Demux : Demux
  Demux1 : Demux  Outputs=2
  Gain : Gain  Gain=d_11
  Gain1 : Gain  Gain=1/(m_RB11+m_A11)
  Gain{8..14} (7 alike) : Gain  Gain=0
  Gain2 : Gain  Gain=d_22
  Gain3 : Gain  Gain=1/(m_RB22+m_A22)
  Gain4 : Gain  Gain=d_33
  Gain5 : Gain  Gain=1/(m_RB33+m_A33)
  Gain6 : Gain  Gain=d_66
  Gain7 : Gain  Gain=1/(m_RB66+m_A66)
  Integrator : Integrator  InitialCondition=u0
  Integrator1 : Integrator  InitialCondition=v0
  Integrator2 : Integrator  InitialCondition=w0
  Integrator3 : Integrator  InitialCondition=r0
  Mux1 : Mux
  Nonlinear damping r : Subsystem
  Nonlinear damping u : Subsystem
  Nonlinear damping v : Subsystem
  Nonlinear damping w : Subsystem
  Sum{,2,4..6,8..10,12} (9 alike) : Sum  Inputs=|+-
  Sum{1,3,7,11,13} (5 alike) : Sum  Inputs=-+|
  Switch{,1..6} (7 alike) : Switch  Criteria=u2 > Threshold
  nu : Outport
  wires:
  Demux1/1 -> [V_x]
  Gain1/1 -> Integrator/1
  Sum/1 -> Gain1/1
  tau/1 -> Demux/1
  Integrator1/1 -> Nonlinear damping v/1(v), Gain2/1, [v], Mux1/2
  Gain3/1 -> Integrator1/1
  Mux1/1 -> nu/1
  Integrator/1 -> Nonlinear damping u/1(u), [u], Mux1/1, Gain/1
  Integrator2/1 -> Gain4/1, Nonlinear damping w/1(w), Mux1/3
  Gain5/1 -> Integrator2/1
  Sum4/1 -> Gain5/1
  Gain2/1 -> Sum2/2
  Sum2/1 -> Gain3/1
  Gain/1 -> Sum/2
  Gain4/1 -> Sum4/2
  Gain6/1 -> Sum6/2
  Demux1/2 -> [V_y]
  [r] -> Current/3(r)
  Integrator3/1 -> [r], Mux1/4, Nonlinear damping r/1(r), Gain6/1
  disturbance/1 -> Demux1/1
  Sum6/1 -> Gain7/1
  Gain7/1 -> Integrator3/1
  psi/1 -> [psi]
  Current/1(-M_A*nu_dot_c-D*nu_c) -> Sum1/1
  [V_y] -> Current/2(V_y)
  [V_x] -> Current/1(V_x)
  [psi] -> Current/4(psi)
  [r] -> Current1/3(r)
  [psi] -> Current1/4(psi)
  [V_x] -> Current1/1(V_x)
  [V_y] -> Current1/2(V_y)
  Current1/1(-M_A*nu_dot_c-D*nu_c) -> Sum3/1
  Constant/1 -> Sum5/2
  Demux/3 -> Sum5/1
  Demux/1 -> Sum7/2
  Sum7/1 -> Sum1/2
  [V_x] -> Coriolis/1(V_x)
  [psi] -> Coriolis/5(psi)
  [r] -> Coriolis/3(r)
  [V_y] -> Coriolis/2(V_y)
  [v] -> Coriolis/4(v)
  [u] -> Coriolis1/4(u)
  [V_y] -> Coriolis1/2(V_y)
  [psi] -> Coriolis1/5(psi)
  [V_x] -> Coriolis1/1(V_x)
  [r] -> Coriolis1/3(r)
  Sum8/1 -> Sum3/2
  Demux/2 -> Sum8/1
  [v] -> Coriolis2/4(v)
  [V_y] -> Coriolis2/2(V_y)
  [psi] -> Coriolis2/5(psi)
  [V_x] -> Coriolis2/1(V_x)
  [u] -> Coriolis2/3(u)
  Demux/4 -> Sum9/1
  Sum10/1 -> Sum6/1
  Sum5/1 -> Sum11/2
  Sum11/1 -> Sum4/1
  Nonlinear damping w/1(D_n(nu_r)nu_r(3)) -> Gain10/1, Switch2/1
  Sum12/1 -> Sum2/1
  Sum1/1 -> Sum13/2
  Sum13/1 -> Sum/1
  Nonlinear damping u/1(D_n(nu_r)nu_r(1)) -> Switch/1, Gain8/1
  [V_x] -> Nonlinear damping u/2(V_x)
  [V_y] -> Nonlinear damping u/3(V_y)
  [psi] -> Nonlinear damping u/4(psi)
  Sum3/1 -> Sum12/1
  Nonlinear damping v/1(D_n(nu_r)nu_r(2)) -> Gain9/1, Switch1/1
  [V_x] -> Nonlinear damping v/2(V_x)
  [V_y] -> Nonlinear damping v/3(V_y)
  [psi] -> Nonlinear damping v/4(psi)
  Sum9/1 -> Sum10/1
  Switch/1 -> Sum13/1
  Switch1/1 -> Sum12/2
  Switch2/1 -> Sum11/1
  Switch3/1 -> Sum10/2
  Constant1/1 -> Switch/2
  Gain8/1 -> Switch/3
  Gain9/1 -> Switch1/3
  Constant2/1 -> Switch1/2
  Gain10/1 -> Switch2/3
  Constant3/1 -> Switch2/2
  Gain11/1 -> Switch3/3
  Constant4/1 -> Switch3/2
  Nonlinear damping r/1(D_n(nu_r)nu_r(6)) -> Switch3/1, Gain11/1
  Switch4/1 -> Sum7/1
  Coriolis/1(C(nu_r)nu_r(1)) -> Switch4/1, Gain12/1
  Constant5/1 -> Switch4/2
  Gain12/1 -> Switch4/3
  Switch5/1 -> Sum8/2
  Gain13/1 -> Switch5/3
  Constant6/1 -> Switch5/2
  Coriolis1/1(C(nu_r)nu_r(2)) -> Switch5/1, Gain13/1
  Coriolis2/1(C(nu_r)nu_r(4)) -> Switch6/1, Gain14/1
  Switch6/1 -> Sum9/2
  Gain14/1 -> Switch6/3
  Constant7/1 -> Switch6/2

== system simulering_ROV_DP_model2/Process plant model/Thruster saturation ==
  tau_unsat : Inport
  Constant : Constant  Value=B_psinv_aug
  Constant1 : Constant  Value=B_aug
  Demux : Demux  Outputs=6
  Matrix Multiply : Product  Multiplication=Matrix(*)
  Matrix Multiply1 : Product  Multiplication=Matrix(*)
  Mux : Mux  Inputs=6
  Saturation{,1..5} (6 alike) : Saturate  UpperLimit=120  LowerLimit=-120
  tau_sat : Outport
  wires:
  tau_unsat/1 -> Matrix Multiply/2
  Constant/1 -> Matrix Multiply/1
  Matrix Multiply/1 -> Demux/1
  Demux/2 -> Saturation1/1
  Demux/1 -> Saturation/1
  Demux/3 -> Saturation2/1
  Demux/4 -> Saturation3/1
  Demux/5 -> Saturation4/1
  Demux/6 -> Saturation5/1
  Saturation/1 -> Mux/1
  Saturation1/1 -> Mux/2
  Saturation2/1 -> Mux/3
  Saturation3/1 -> Mux/4
  Saturation4/1 -> Mux/5
  Saturation5/1 -> Mux/6
  Mux/1 -> Matrix Multiply1/2
  Constant1/1 -> Matrix Multiply1/1
  Matrix Multiply1/1 -> tau_sat/1

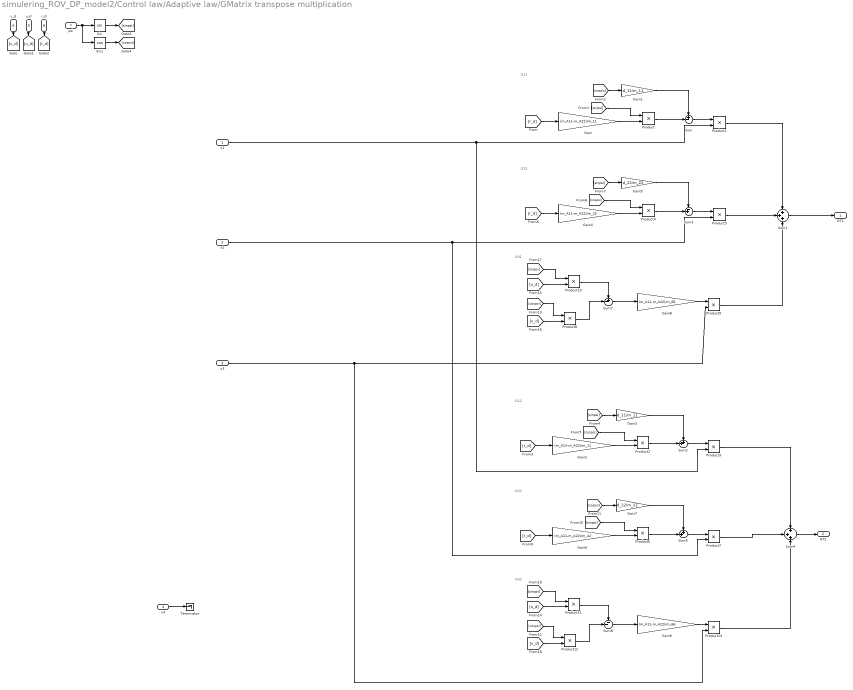
== system simulering_ROV_DP_model2/Control law/Adaptive law/GMatrix transpose multiplication ==
  note: G31
  note: G22
  note: G21
  note: G12
  note: G11
  note: G32
  x1 : Inport
  x2 : Inport  Port=2
  x3 : Inport  Port=3
  x4 : Inport  Port=4
  u_d : Inport  Port=5
  v_d : Inport  Port=6
  psi : Inport  Port=7
  r_d : Inport  Port=8
  Gain : Gain  Gain=(m_A11-m_A22)/m_11
  Gain1 : Gain  Gain=d_11/m_11
  Gain2 : Gain  Gain=(m_A11-m_A22)/m_11
  Gain3 : Gain  Gain=d_11/m_11
  Gain4 : Gain  Gain=(m_A11-m_A22)/m_22
  Gain5 : Gain  Gain=d_22/m_22
  Gain6 : Gain  Gain=(m_A11-m_A22)/m_22
  Gain7 : Gain  Gain=d_22/m_22
  Gain8 : Gain  Gain=(m_A11-m_A22)/m_66
  Gain9 : Gain  Gain=(m_A11-m_A22)/m_66
  Product{,1..13} (14 alike) : Product
  Sin : Trigonometry
  Sin1 : Trigonometry  Operator=cos
  Sum : Sum  Inputs=+-|
  Sum1 : Sum  Inputs=+++
  Sum2 : Sum  Inputs=++|
  Sum3 : Sum  Inputs=-+|
  Sum4 : Sum  Inputs=+++
  Sum5 : Sum  Inputs=++|
  Sum7 : Sum  Inputs=+-|
  Sum8 : Sum  Inputs=--|
  Terminator : Terminator
  GT1 : Outport
  GT2 : Outport  Port=2
  wires:
  v_d/1 -> [v_d]
  u_d/1 -> [u_d]
  r_d/1 -> [r_d]
  psi/1 -> Sin1/1, Sin/1
  Sin/1 -> [sinpsi]
  Sin1/1 -> [cospsi]
  Product1/1 -> Sum1/1
  Sum/1 -> Product1/1
  Product/1 -> Sum/2
  [r_d] -> Gain/1
  Gain/1 -> Product/2
  [sinpsi] -> Product/1
  [cospsi] -> Gain1/1
  Gain1/1 -> Sum/1
  Sum1/1 -> GT1/1
  Sum2/1 -> Product3/1
  Product2/1 -> Sum2/2
  [r_d] -> Gain2/1
  Gain2/1 -> Product2/2
  [cospsi] -> Product2/1
  [sinpsi] -> Gain3/1
  Gain3/1 -> Sum2/1
  x1/1 -> Product3/2, Product1/2
  Sum3/1 -> Product5/1
  Product4/1 -> Sum3/2
  [r_d] -> Gain4/1
  Gain4/1 -> Product4/2
  [cospsi] -> Product4/1
  [sinpsi] -> Gain5/1
  Gain5/1 -> Sum3/1
  Sum5/1 -> Product7/1
  Product6/1 -> Sum5/2
  [r_d] -> Gain6/1
  Gain6/1 -> Product6/2
  [sinpsi] -> Product6/1
  [cospsi] -> Gain7/1
  Gain7/1 -> Sum5/1
  Sum7/1 -> Gain8/1
  [u_d] -> Product10/2
  [sinpsi] -> Product10/1
  [v_d] -> Product8/2
  [cospsi] -> Product8/1
  Product8/1 -> Sum7/2
  Product10/1 -> Sum7/1
  Gain8/1 -> Product9/1
  Sum8/1 -> Gain9/1
  Product12/1 -> Sum8/2
  [u_d] -> Product11/2
  [sinpsi] -> Product11/1
  [v_d] -> Product12/2
  Gain9/1 -> Product13/1
  [cospsi] -> Product12/1
  Product11/1 -> Sum8/1
  Product5/1 -> Sum1/2
  Product9/1 -> Sum1/3
  Sum4/1 -> GT2/1
  Product7/1 -> Sum4/2
  Product3/1 -> Sum4/1
  Product13/1 -> Sum4/3
  x2/1 -> Product7/2, Product5/2
  x3/1 -> Product13/2, Product9/2
  x4/1 -> Terminator/1

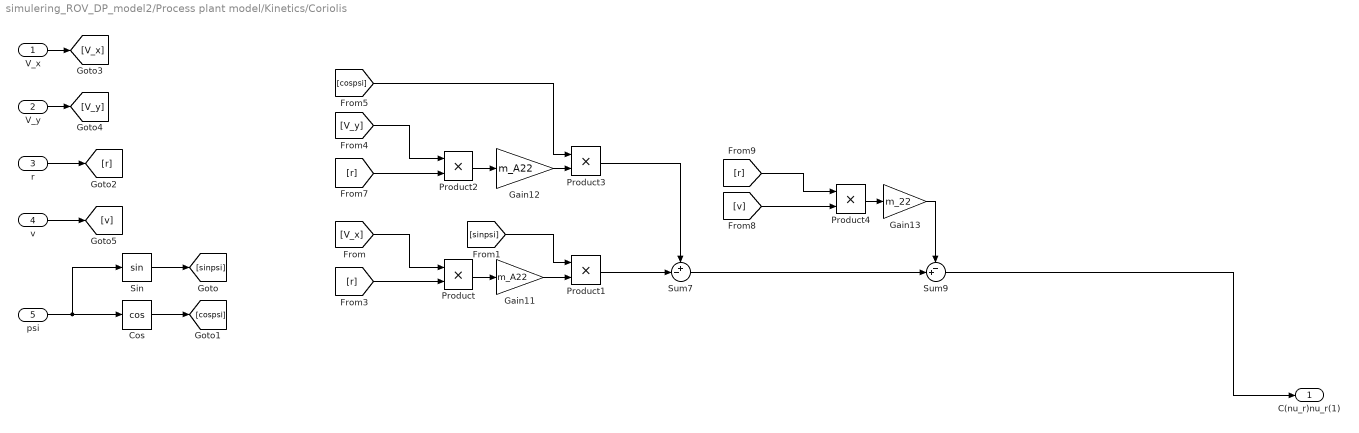
== system simulering_ROV_DP_model2/Process plant model/Kinetics/Coriolis ==
  V_x : Inport
  V_y : Inport  Port=2
  r : Inport  Port=3
  v : Inport  Port=4
  psi : Inport  Port=5
  Cos : Trigonometry  Operator=cos
  Gain11 : Gain  Gain=m_A22
  Gain12 : Gain  Gain=m_A22
  Gain13 : Gain  Gain=m_22
  Product{,1..4} (5 alike) : Product
  Sin : Trigonometry
  Sum7 : Sum  Inputs=+-|
  Sum9 : Sum  Inputs=-+|
  C(nu_r)nu_r(1) : Outport
  wires:
  Gain11/1 -> Product1/2
  Product2/1 -> Gain12/1
  [cospsi] -> Product3/1
  [r] -> Product2/2
  [v] -> Product4/2
  Product4/1 -> Gain13/1
  [V_x] -> Product/1
  Product3/1 -> Sum7/1
  Gain12/1 -> Product3/2
  Product/1 -> Gain11/1
  [V_y] -> Product2/1
  [r] -> Product/2
  Product1/1 -> Sum7/2
  [sinpsi] -> Product1/1
  Sum7/1 -> Sum9/2
  [r] -> Product4/1
  Sum9/1 -> C(nu_r)nu_r(1)/1
  psi/1 -> Sin/1, Cos/1
  Sin/1 -> [sinpsi]
  Cos/1 -> [cospsi]
  r/1 -> [r]
  V_x/1 -> [V_x]
  V_y/1 -> [V_y]
  v/1 -> [v]
  Gain13/1 -> Sum9/1

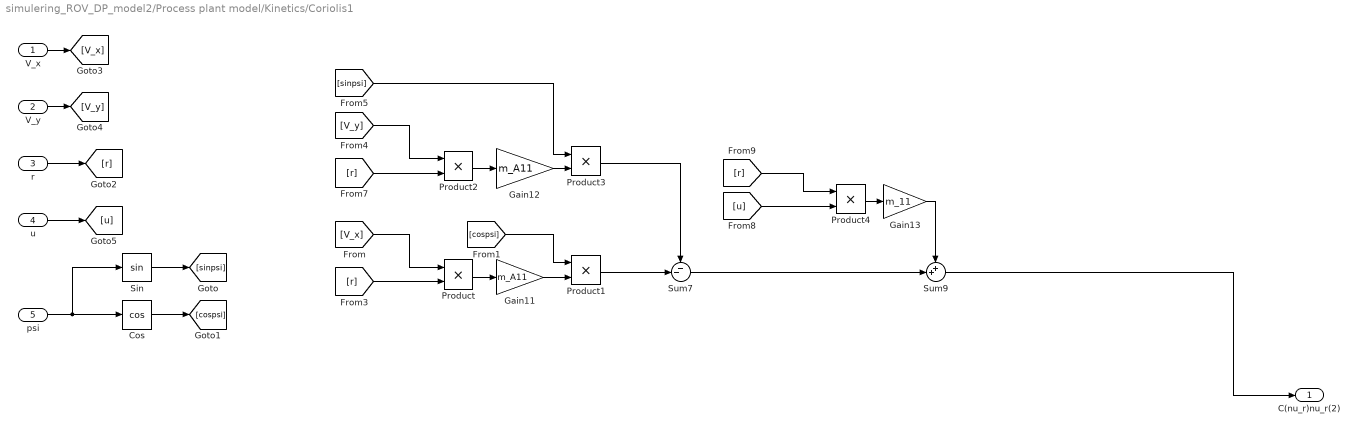
== system simulering_ROV_DP_model2/Process plant model/Kinetics/Coriolis1 ==
  V_x : Inport
  V_y : Inport  Port=2
  r : Inport  Port=3
  u : Inport  Port=4
  psi : Inport  Port=5
  Cos : Trigonometry  Operator=cos
  Gain11 : Gain  Gain=m_A11
  Gain12 : Gain  Gain=m_A11
  Gain13 : Gain  Gain=m_11
  Product{,1..4} (5 alike) : Product
  Sin : Trigonometry
  Sum7 : Sum  Inputs=--|
  Sum9 : Sum  Inputs=++|
  C(nu_r)nu_r(2) : Outport
  wires:
  Gain11/1 -> Product1/2
  Product2/1 -> Gain12/1
  [sinpsi] -> Product3/1
  [r] -> Product2/2
  [u] -> Product4/2
  Product4/1 -> Gain13/1
  [V_x] -> Product/1
  Product3/1 -> Sum7/1
  Gain12/1 -> Product3/2
  Product/1 -> Gain11/1
  [V_y] -> Product2/1
  [r] -> Product/2
  Product1/1 -> Sum7/2
  [cospsi] -> Product1/1
  Sum7/1 -> Sum9/2
  [r] -> Product4/1
  Sum9/1 -> C(nu_r)nu_r(2)/1
  psi/1 -> Sin/1, Cos/1
  Sin/1 -> [sinpsi]
  Cos/1 -> [cospsi]
  r/1 -> [r]
  V_x/1 -> [V_x]
  V_y/1 -> [V_y]
  u/1 -> [u]
  Gain13/1 -> Sum9/1

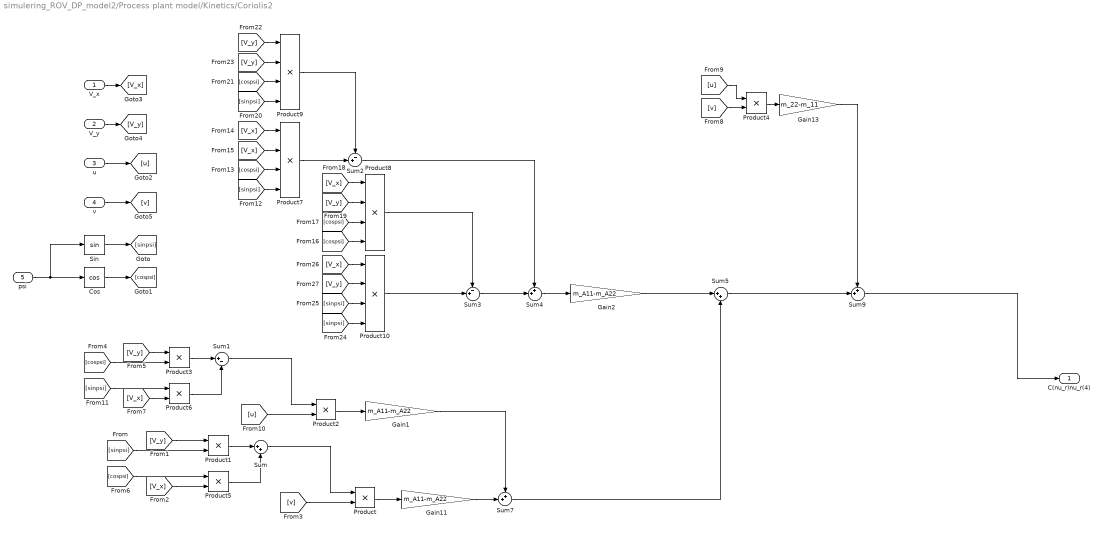
== system simulering_ROV_DP_model2/Process plant model/Kinetics/Coriolis2 ==
  V_x : Inport
  V_y : Inport  Port=2
  u : Inport  Port=3
  v : Inport  Port=4
  psi : Inport  Port=5
  Cos : Trigonometry  Operator=cos
  Gain1 : Gain  Gain=m_A11-m_A22
  Gain11 : Gain  Gain=m_A11-m_A22
  Gain13 : Gain  Gain=m_22-m_11
  Gain2 : Gain  Gain=m_A11-m_A22
  Product{,1..6} (7 alike) : Product
  Product{7..10} (4 alike) : Product  Inputs=4
  Sin : Trigonometry
  Sum : Sum  Inputs=|++
  Sum1 : Sum  Inputs=|+-
  Sum2 : Sum  Inputs=-+|
  Sum3 : Sum  Inputs=-+|
  Sum4 : Sum  Inputs=++|
  Sum5 : Sum  Inputs=|++
  Sum7 : Sum  Inputs=++|
  Sum9 : Sum  Inputs=++|
  C(nu_r)nu_r(4) : Outport
  wires:
  [v] -> Product4/2
  Product4/1 -> Gain13/1
  Product/1 -> Gain11/1
  [v] -> Product/2
  Gain11/1 -> Sum7/2
  [u] -> Product4/1
  Sum9/1 -> C(nu_r)nu_r(4)/1
  psi/1 -> Sin/1, Cos/1
  Sin/1 -> [sinpsi]
  Cos/1 -> [cospsi]
  u/1 -> [u]
  V_x/1 -> [V_x]
  V_y/1 -> [V_y]
  v/1 -> [v]
  Gain13/1 -> Sum9/1
  [V_y] -> Product1/1
  [V_x] -> Product5/2
  Product1/1 -> Sum/1
  Product5/1 -> Sum/2
  Sum/1 -> Product/1
  [sinpsi] -> Product1/2
  [cospsi] -> Product5/1
  Product2/1 -> Gain1/1
  [u] -> Product2/2
  [V_x] -> Product6/2
  Sum1/1 -> Product2/1
  [cospsi] -> Product3/2
  [V_y] -> Product3/1
  [sinpsi] -> Product6/1
  Product3/1 -> Sum1/1
  Product6/1 -> Sum1/2
  Gain1/1 -> Sum7/1
  [sinpsi] -> Product7/4
  [cospsi] -> Product7/3
  [V_x] -> Product7/1
  [V_x] -> Product7/2
  [sinpsi] -> Product9/4
  [V_y] -> Product9/1
  [cospsi] -> Product9/3
  [V_y] -> Product9/2
  Product7/1 -> Sum2/2
  Product9/1 -> Sum2/1
  [V_y] -> Product8/2
  [cospsi] -> Product8/3
  [V_x] -> Product8/1
  Product8/1 -> Sum3/1
  [cospsi] -> Product8/4
  [V_y] -> Product10/2
  [sinpsi] -> Product10/3
  [V_x] -> Product10/1
  [sinpsi] -> Product10/4
  Product10/1 -> Sum3/2
  Sum3/1 -> Sum4/2
  Sum2/1 -> Sum4/1
  Sum4/1 -> Gain2/1
  Sum7/1 -> Sum5/2
  Sum5/1 -> Sum9/2
  Gain2/1 -> Sum5/1

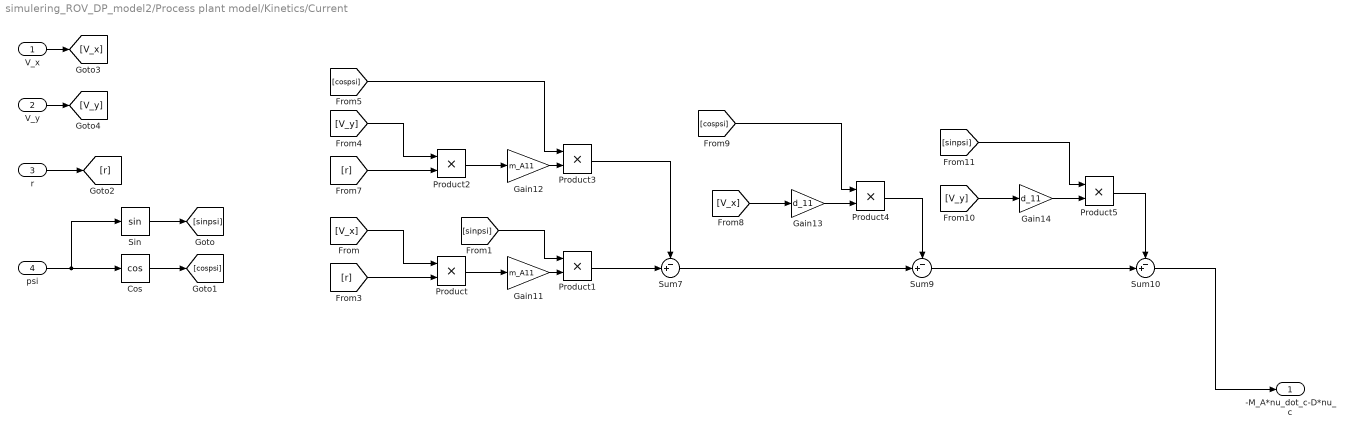
== system simulering_ROV_DP_model2/Process plant model/Kinetics/Current ==
  V_x : Inport
  V_y : Inport  Port=2
  r : Inport  Port=3
  psi : Inport  Port=4
  Cos : Trigonometry  Operator=cos
  Gain11 : Gain  Gain=m_A11
  Gain12 : Gain  Gain=m_A11
  Gain13 : Gain  Gain=d_11
  Gain14 : Gain  Gain=d_11
  Product{,1..5} (6 alike) : Product
  Sin : Trigonometry
  Sum10 : Sum  Inputs=-+|
  Sum7 : Sum  Inputs=-+|
  Sum9 : Sum  Inputs=-+|
  -M_A*nu_dot_c-D*nu_c : Outport
  wires:
  Gain11/1 -> Product1/2
  Product2/1 -> Gain12/1
  [cospsi] -> Product3/1
  [r] -> Product2/2
  Gain13/1 -> Product4/2
  Product4/1 -> Sum9/1
  [V_x] -> Product/1
  Product3/1 -> Sum7/1
  Gain12/1 -> Product3/2
  Product/1 -> Gain11/1
  [V_y] -> Product2/1
  [r] -> Product/2
  Product1/1 -> Sum7/2
  [sinpsi] -> Product1/1
  Gain14/1 -> Product5/2
  [sinpsi] -> Product5/1
  Sum7/1 -> Sum9/2
  [cospsi] -> Product4/1
  [V_y] -> Gain14/1
  [V_x] -> Gain13/1
  Product5/1 -> Sum10/1
  Sum9/1 -> Sum10/2
  Sum10/1 -> -M_A*nu_dot_c-D*nu_c/1
  psi/1 -> Sin/1, Cos/1
  Sin/1 -> [sinpsi]
  Cos/1 -> [cospsi]
  r/1 -> [r]
  V_x/1 -> [V_x]
  V_y/1 -> [V_y]

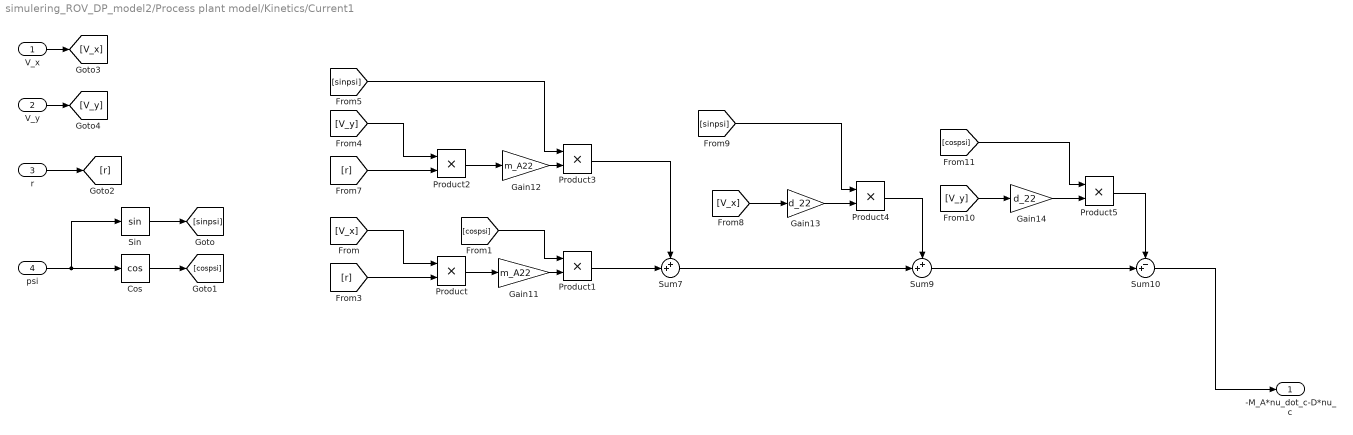
== system simulering_ROV_DP_model2/Process plant model/Kinetics/Current1 ==
  V_x : Inport
  V_y : Inport  Port=2
  r : Inport  Port=3
  psi : Inport  Port=4
  Cos : Trigonometry  Operator=cos
  Gain11 : Gain  Gain=m_A22
  Gain12 : Gain  Gain=m_A22
  Gain13 : Gain  Gain=d_22
  Gain14 : Gain  Gain=d_22
  Product{,1..5} (6 alike) : Product
  Sin : Trigonometry
  Sum10 : Sum  Inputs=-+|
  Sum7 : Sum  Inputs=++|
  Sum9 : Sum  Inputs=++|
  -M_A*nu_dot_c-D*nu_c : Outport
  wires:
  Gain11/1 -> Product1/2
  Product2/1 -> Gain12/1
  [sinpsi] -> Product3/1
  [r] -> Product2/2
  Gain13/1 -> Product4/2
  Product4/1 -> Sum9/1
  [V_x] -> Product/1
  Product3/1 -> Sum7/1
  Gain12/1 -> Product3/2
  Product/1 -> Gain11/1
  [V_y] -> Product2/1
  [r] -> Product/2
  Product1/1 -> Sum7/2
  [cospsi] -> Product1/1
  Gain14/1 -> Product5/2
  [cospsi] -> Product5/1
  Sum7/1 -> Sum9/2
  [sinpsi] -> Product4/1
  [V_y] -> Gain14/1
  [V_x] -> Gain13/1
  Product5/1 -> Sum10/1
  Sum9/1 -> Sum10/2
  Sum10/1 -> -M_A*nu_dot_c-D*nu_c/1
  psi/1 -> Sin/1, Cos/1
  Sin/1 -> [sinpsi]
  Cos/1 -> [cospsi]
  r/1 -> [r]
  V_x/1 -> [V_x]
  V_y/1 -> [V_y]

== system simulering_ROV_DP_model2/Process plant model/Kinetics/Nonlinear damping r ==
  r : Inport
  Abs : Abs
  Gain : Gain  Gain=d_n66
  Product : Product
  To Workspace : ToWorkspace  VariableName=r_relative_vel  SaveFormat=Structure With Time  SampleTime=-1
  D_n(nu_r)nu_r(6) : Outport
  wires:
  Abs/1 -> Gain/1
  Product/1 -> D_n(nu_r)nu_r(6)/1
  Gain/1 -> Product/1
  r/1 -> To Workspace/1, Abs/1, Product/2
